simulink model "lab1"  (R2018a)
settings: Solver=VariableStepAuto  StartTime=0.0  StopTime=100  RelTol=1e-3
settings Model: Creator=Yan Tszyafen  LastModifiedBy=Yan Tszyafen

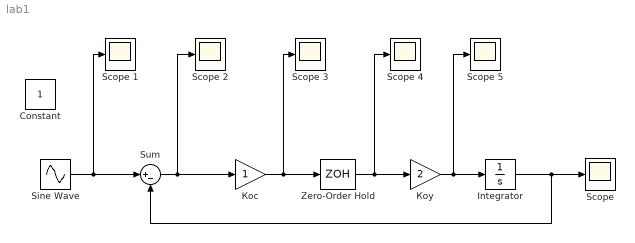
== system lab1 ==
  Constant : Constant
  Integrator : Integrator
  Scope {,1..5} (6 alike) : Scope
  Sine Wave : Sin  SampleTime=0
  Sum : Sum  Inputs=|+-
  Zero-Order Hold : ZeroOrderHold
  Кос : Gain
  Коу : Gain  Gain=2
  wires:
  Sine Wave/1 -> Scope 1/1, Sum/1
  Sum/1 -> Scope 2/1, Кос/1
  Кос/1 -> Scope 3/1, Zero-Order Hold/1
  Zero-Order Hold/1 -> Scope 4/1, Коу/1
  Коу/1 -> Scope 5/1, Integrator/1
  Integrator/1 -> Sum/2, "Scope "/1
